simulink model "model_cnn"  (R2020a)
settings: Solver=VariableStepAuto  StartTime=0.0  StopTime=1e6/fs  RelTol=1e-3
PreLoadFcn:
  | setup_imports;
  | %dense2_numerictype = fixdt(1,18,10);
  | %conv1_numerictype = fixdt(1,18,21);
InitFcn:
  | % Intermediate signal dimensions
  | input_dim = [1, 2, 128];
  | layer1_dim = hInterConvLayerDims([1,3,1,64],input_dim,1); % dims : [C,H,W]
  | layer2_dim = hInterConvLayerDims([2,3,64,16],layer1_dim,1);% dims : [C,H,W]
  | layer3_dim = [1,128];
  | 
  | % Conv Layer 1 dimensions
  | conv1_dims = struct(...
  |     'input_dim',    input_dim,...       input_dim = C,H,W
  |     'filter_dim',   [1, 3, 1, 64],...  filter_dim = K,J,C,N
  |     'stride',       1,...
  |     'row_output',   3,...
  |     'output_dim',   layer1_dim);
  | 
  | % Conv Layer 2 dimensions
  | conv2_dims = struct(...
  |     'input_dim',    layer1_dim,...      input = C,H.W
  |     'filter_dim',   [2, 3, 64, 16],...  filter_dim = K,J,C,N
  |     'stride',       1,...
  |     'row_output',   2*3*64,...
  |     'output_dim',   layer2_dim);
  | 
  | % Dense Layer 1 dimensions
  | dense1_dims = struct(...
  |     'input_dim',    layer2_dim,...      input = C,H,W
  |     'weight_dim',   [1984, 128],...     weight_dim = H,W
  |     'output_dim',   layer3_dim);
  | 
  | % Load saved weights and input
  | setup_imports;
  | 
  | fs = 128e6;
  | fs_axi = 100e6;
  | R = 32;
values from neighbouring files (symbols this model uses):
  datatypeInput = X_test.numerictype    [setup_imports.m]
  gemm_wconv1 = fi(hInterleaveFilters(Wconv1),1,16)    [setup_imports.m]
  gemm_wconv2 = fi(hInterleaveFilters(Wconv2),1,16)    [setup_imports.m]
  wdense1 = fi(Wdense1,1,16)    [setup_imports.m]
  wdense2 = fi(Wdense2,1,16)    [setup_imports.m]
undefined symbols (not defined in the file or in its folder): ltehdlRAMinitPO2
libraries: hdlsllib x1022, dspsigops x3, dspsrcs4 x2
(part 2 of 23)

== system model_cnn/HDL CNN Model/Conv Layer 2/Vector Slice Selection ==
  frameIn : Inport
  validIn : Inport  Port=2
  Frame Slicer : MATLAB Function  TreatAsAtomicUnit=on
  Frame Slicer1 : MATLAB Function  TreatAsAtomicUnit=on
  Frame Slicer2 : MATLAB Function  TreatAsAtomicUnit=on
  Frame Slicer3 : MATLAB Function  TreatAsAtomicUnit=on
  HDL Counter : hdlsllib/Sources/HDL Counter  CountType=Count limited  CountInit=0  CountStep=1  CountMax=3  CountFromType=Initial value  CountFrom=0  CountResetPort=off  CountLoadPort=off  CountEnbPort=on  CountDirPort=off  CountDataType=Unsigned  CountWordLen=2  CountFracLen=0  CountSampTime=1
  Multiport Switch : MultiPortSwitch  DataPortOrder=Zero-based contiguous  Inputs=4  DiagnosticForDefault=None  zeroidx=on
  frameOut : Outport
  validOut : Outport  Port=2
  wires:
  frameIn/1 -> Frame Slicer/1(frameIn), Frame Slicer3/1(frameIn), Frame Slicer2/1(frameIn), Frame Slicer1/1(frameIn)
  validIn/1 -> validOut/1, HDL Counter/1
  HDL Counter/1 -> Multiport Switch/1
  Frame Slicer/1(slicedFrame) -> Multiport Switch/2
  Frame Slicer1/1(slicedFrame) -> Multiport Switch/3
  Frame Slicer2/1(slicedFrame) -> Multiport Switch/4
  Frame Slicer3/1(slicedFrame) -> Multiport Switch/5
  Multiport Switch/1 -> frameOut/1

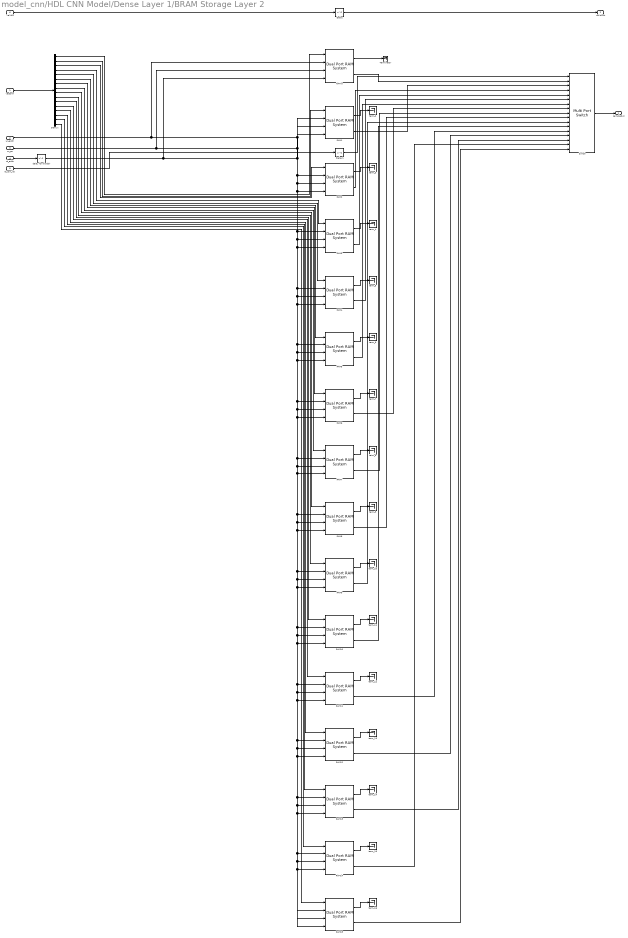
== system model_cnn/HDL CNN Model/Dense Layer 1/BRAM Storage Layer 2 ==
  vectorIn : Inport
  wr_addr : Inport  Port=2
  wr_en : Inport  Port=3
  rd_addr : Inport  Port=4
  rd_row_idx : Inport  Port=5
  validIn : Inport  Port=6
  Delay : Delay
  Delay1 : Delay
  Demux : Demux  Outputs=16
  RAM 0 : hdlsllib/HDL RAMs/Dual Port RAM System  RAMType=Dual port  WriteOutputValue=New data  RAMInitialValue=0  SimulateUsing=Code generation
      settings: SourceProductBaseCode=SL
  RAM{1..15} (15 alike) : hdlsllib/HDL RAMs/Dual Port RAM System  RAMType=Dual port  WriteOutputValue=New data  RAMInitialValue=0  SimulateUsing=Code generation
      settings: SourceProductBaseCode=SL
  Switch : MultiPortSwitch  DataPortOrder=Zero-based contiguous  Inputs=16  zeroidx=on
  Terminator : Terminator
  delay for rd addr : Delay  DelayLength=1
  term_{2..16} (15 alike) : Terminator
  sampleOut : Outport
  validOut : Outport  Port=2
  wires:
  vectorIn/1 -> Demux/1  "vectorIn"
  Demux/1 -> RAM 0/1
  Switch/1 -> sampleOut/1  "fff_sampleOut"
  wr_addr/1 -> RAM15/2, RAM14/2, RAM13/2, RAM12/2, RAM11/2, RAM10/2, RAM9/2, RAM8/2, RAM7/2, RAM6/2, RAM5/2, RAM4/2, RAM3/2, RAM2/2, RAM1/2, RAM 0/2  "wr_addr"
  RAM 0/1 -> Terminator/1
  RAM 0/2 -> Switch/2  "ram_out"
  validIn/1 -> Delay/1  "vvv valid"
  Delay/1 -> validOut/1  "fff_valid"
  wr_en/1 -> RAM15/3, RAM14/3, RAM13/3, RAM12/3, RAM11/3, RAM10/3, RAM9/3, RAM8/3, RAM7/3, RAM6/3, RAM5/3, RAM4/3, RAM3/3, RAM2/3, RAM1/3, RAM 0/3  "wr_en"
  rd_addr/1 -> delay for rd addr/1  "fff_rd_addr"
  Demux/2 -> RAM1/1
  RAM1/2 -> Switch/3  "fff_rd_row_2"
  RAM1/1 -> term_2/1
  Demux/3 -> RAM2/1
  RAM2/2 -> Switch/4
  RAM2/1 -> term_3/1
  Demux/4 -> RAM3/1
  RAM3/2 -> Switch/5
  RAM3/1 -> term_4/1
  Demux/5 -> RAM4/1
  RAM4/2 -> Switch/6
  RAM4/1 -> term_5/1
  Demux/6 -> RAM5/1  "vvv"
  RAM5/2 -> Switch/7
  RAM5/1 -> term_6/1
  Demux/7 -> RAM6/1
  RAM6/2 -> Switch/8
  RAM6/1 -> term_7/1
  Demux/8 -> RAM7/1
  RAM7/2 -> Switch/9
  RAM7/1 -> term_8/1
  Demux/9 -> RAM8/1
  RAM8/2 -> Switch/10
  RAM8/1 -> term_9/1
  Demux/10 -> RAM9/1
  RAM9/2 -> Switch/11
  RAM9/1 -> term_10/1
  Demux/11 -> RAM10/1
  RAM10/2 -> Switch/12
  RAM10/1 -> term_11/1
  Demux/12 -> RAM11/1
  RAM11/2 -> Switch/13
  RAM11/1 -> term_12/1
  Demux/13 -> RAM12/1
  RAM12/2 -> Switch/14
  RAM12/1 -> term_13/1
  Demux/14 -> RAM13/1
  RAM13/2 -> Switch/15
  RAM13/1 -> term_14/1
  Demux/15 -> RAM14/1
  RAM14/2 -> Switch/16
  RAM14/1 -> term_15/1
  Demux/16 -> RAM15/1
  RAM15/2 -> Switch/17  "valueOut"
  RAM15/1 -> term_16/1
  rd_row_idx/1 -> Delay1/1
  Delay1/1 -> Switch/1  "fff_rd_row"
  delay for rd addr/1 -> RAM15/4, RAM14/4, RAM13/4, RAM12/4, RAM11/4, RAM10/4, RAM9/4, RAM8/4, RAM7/4, RAM6/4, RAM5/4, RAM4/4, RAM3/4, RAM2/4, RAM1/4, RAM 0/4

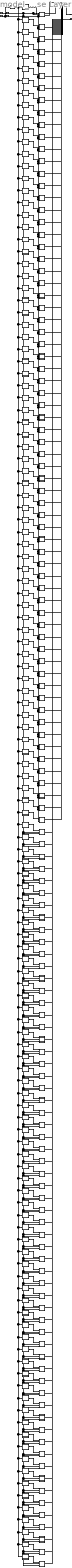
== system model_cnn/HDL CNN Model/Dense Layer 1/Dense Layer 1 ==
  dataIn : Inport
  valid : Inport  Port=2
  Delay : Delay  DelayLength=1
  Delay1 : Delay  DelayLength=1
  HDL Counter : hdlsllib/Sources/HDL Counter  CountType=Count limited  CountInit=0  CountStep=1  CountMax=1984-1  CountFromType=Initial value  CountFrom=0  CountResetPort=off  CountLoadPort=off  CountEnbPort=on  CountDirPort=off  CountDataType=Unsigned  CountWordLen=ceil(log2(1984))  CountFracLen=0  CountSampTime=1
  Vector Concatenate : Concatenate  NumInputs=128
  Weight Storage 0 : Subsystem  mask{dim=1}
      mask prompts: dim "Filter Selection"
  Weight Storage1 : Subsystem  mask{dim=2}
      mask prompts: dim "Filter Selection"
  Weight Storage10 : Subsystem  mask{dim=11}
      mask prompts: dim "Filter Selection"
  Weight Storage100 : Subsystem  mask{dim=101}
      mask prompts: dim "Filter Selection"
  Weight Storage101 : Subsystem  mask{dim=102}
      mask prompts: dim "Filter Selection"
  Weight Storage102 : Subsystem  mask{dim=103}
      mask prompts: dim "Filter Selection"
  Weight Storage103 : Subsystem  mask{dim=104}
      mask prompts: dim "Filter Selection"
  Weight Storage104 : Subsystem  mask{dim=105}
      mask prompts: dim "Filter Selection"
  Weight Storage105 : Subsystem  mask{dim=106}
      mask prompts: dim "Filter Selection"
  Weight Storage106 : Subsystem  mask{dim=107}
      mask prompts: dim "Filter Selection"
  Weight Storage107 : Subsystem  mask{dim=108}
      mask prompts: dim "Filter Selection"
  Weight Storage108 : Subsystem  mask{dim=109}
      mask prompts: dim "Filter Selection"
  Weight Storage109 : Subsystem  mask{dim=110}
      mask prompts: dim "Filter Selection"
  Weight Storage11 : Subsystem  mask{dim=12}
      mask prompts: dim "Filter Selection"
  Weight Storage110 : Subsystem  mask{dim=111}
      mask prompts: dim "Filter Selection"
  Weight Storage111 : Subsystem  mask{dim=112}
      mask prompts: dim "Filter Selection"
  Weight Storage112 : Subsystem  mask{dim=113}
      mask prompts: dim "Filter Selection"
  Weight Storage113 : Subsystem  mask{dim=114}
      mask prompts: dim "Filter Selection"
  Weight Storage114 : Subsystem  mask{dim=115}
      mask prompts: dim "Filter Selection"
  Weight Storage115 : Subsystem  mask{dim=116}
      mask prompts: dim "Filter Selection"
  Weight Storage116 : Subsystem  mask{dim=117}
      mask prompts: dim "Filter Selection"
  Weight Storage117 : Subsystem  mask{dim=118}
      mask prompts: dim "Filter Selection"
  Weight Storage118 : Subsystem  mask{dim=119}
      mask prompts: dim "Filter Selection"
  Weight Storage119 : Subsystem  mask{dim=120}
      mask prompts: dim "Filter Selection"
  Weight Storage12 : Subsystem  mask{dim=13}
      mask prompts: dim "Filter Selection"
  Weight Storage120 : Subsystem  mask{dim=121}
      mask prompts: dim "Filter Selection"
  Weight Storage121 : Subsystem  mask{dim=122}
      mask prompts: dim "Filter Selection"
  Weight Storage122 : Subsystem  mask{dim=123}
      mask prompts: dim "Filter Selection"
  Weight Storage123 : Subsystem  mask{dim=124}
      mask prompts: dim "Filter Selection"
  Weight Storage124 : Subsystem  mask{dim=125}
      mask prompts: dim "Filter Selection"
  Weight Storage125 : Subsystem  mask{dim=126}
      mask prompts: dim "Filter Selection"
  Weight Storage126 : Subsystem  mask{dim=127}
      mask prompts: dim "Filter Selection"
  Weight Storage127 : Subsystem  mask{dim=128}
      mask prompts: dim "Filter Selection"
  Weight Storage13 : Subsystem  mask{dim=14}
      mask prompts: dim "Filter Selection"
  Weight Storage14 : Subsystem  mask{dim=15}
      mask prompts: dim "Filter Selection"
  Weight Storage15 : Subsystem  mask{dim=16}
      mask prompts: dim "Filter Selection"
  Weight Storage16 : Subsystem  mask{dim=17}
      mask prompts: dim "Filter Selection"
  Weight Storage17 : Subsystem  mask{dim=18}
      mask prompts: dim "Filter Selection"
  Weight Storage18 : Subsystem  mask{dim=19}
      mask prompts: dim "Filter Selection"
  Weight Storage19 : Subsystem  mask{dim=20}
      mask prompts: dim "Filter Selection"
  Weight Storage2 : Subsystem  mask{dim=3}
      mask prompts: dim "Filter Selection"
  Weight Storage20 : Subsystem  mask{dim=21}
      mask prompts: dim "Filter Selection"
  Weight Storage21 : Subsystem  mask{dim=22}
      mask prompts: dim "Filter Selection"
  Weight Storage22 : Subsystem  mask{dim=23}
      mask prompts: dim "Filter Selection"
  Weight Storage23 : Subsystem  mask{dim=24}
      mask prompts: dim "Filter Selection"
  Weight Storage24 : Subsystem  mask{dim=25}
      mask prompts: dim "Filter Selection"
  Weight Storage25 : Subsystem  mask{dim=26}
      mask prompts: dim "Filter Selection"
  Weight Storage26 : Subsystem  mask{dim=27}
      mask prompts: dim "Filter Selection"
  Weight Storage27 : Subsystem  mask{dim=28}
      mask prompts: dim "Filter Selection"
  Weight Storage28 : Subsystem  mask{dim=29}
      mask prompts: dim "Filter Selection"
  Weight Storage29 : Subsystem  mask{dim=30}
      mask prompts: dim "Filter Selection"
  Weight Storage3 : Subsystem  mask{dim=4}
      mask prompts: dim "Filter Selection"
  Weight Storage30 : Subsystem  mask{dim=31}
      mask prompts: dim "Filter Selection"
  Weight Storage31 : Subsystem  mask{dim=32}
      mask prompts: dim "Filter Selection"
  Weight Storage32 : Subsystem  mask{dim=33}
      mask prompts: dim "Filter Selection"
  Weight Storage33 : Subsystem  mask{dim=34}
      mask prompts: dim "Filter Selection"
  Weight Storage34 : Subsystem  mask{dim=35}
      mask prompts: dim "Filter Selection"
  Weight Storage35 : Subsystem  mask{dim=36}
      mask prompts: dim "Filter Selection"
  Weight Storage36 : Subsystem  mask{dim=37}
      mask prompts: dim "Filter Selection"
  Weight Storage37 : Subsystem  mask{dim=38}
      mask prompts: dim "Filter Selection"
  Weight Storage38 : Subsystem  mask{dim=39}
      mask prompts: dim "Filter Selection"
  Weight Storage39 : Subsystem  mask{dim=40}
      mask prompts: dim "Filter Selection"
  Weight Storage4 : Subsystem  mask{dim=5}
      mask prompts: dim "Filter Selection"
  Weight Storage40 : Subsystem  mask{dim=41}
      mask prompts: dim "Filter Selection"
  Weight Storage41 : Subsystem  mask{dim=42}
      mask prompts: dim "Filter Selection"
  Weight Storage42 : Subsystem  mask{dim=43}
      mask prompts: dim "Filter Selection"
  Weight Storage43 : Subsystem  mask{dim=44}
      mask prompts: dim "Filter Selection"
  Weight Storage44 : Subsystem  mask{dim=45}
      mask prompts: dim "Filter Selection"
  Weight Storage45 : Subsystem  mask{dim=46}
      mask prompts: dim "Filter Selection"
  Weight Storage46 : Subsystem  mask{dim=47}
      mask prompts: dim "Filter Selection"
  Weight Storage47 : Subsystem  mask{dim=48}
      mask prompts: dim "Filter Selection"
  Weight Storage48 : Subsystem  mask{dim=49}
      mask prompts: dim "Filter Selection"
  Weight Storage49 : Subsystem  mask{dim=50}
      mask prompts: dim "Filter Selection"
  Weight Storage5 : Subsystem  mask{dim=6}
      mask prompts: dim "Filter Selection"
  Weight Storage50 : Subsystem  mask{dim=51}
      mask prompts: dim "Filter Selection"
  Weight Storage51 : Subsystem  mask{dim=52}
      mask prompts: dim "Filter Selection"
  Weight Storage52 : Subsystem  mask{dim=53}
      mask prompts: dim "Filter Selection"
  Weight Storage53 : Subsystem  mask{dim=54}
      mask prompts: dim "Filter Selection"
  Weight Storage54 : Subsystem  mask{dim=55}
      mask prompts: dim "Filter Selection"
  Weight Storage55 : Subsystem  mask{dim=56}
      mask prompts: dim "Filter Selection"
  Weight Storage56 : Subsystem  mask{dim=57}
      mask prompts: dim "Filter Selection"
  Weight Storage57 : Subsystem  mask{dim=58}
      mask prompts: dim "Filter Selection"
  Weight Storage58 : Subsystem  mask{dim=59}
      mask prompts: dim "Filter Selection"
  Weight Storage59 : Subsystem  mask{dim=60}
      mask prompts: dim "Filter Selection"
  Weight Storage6 : Subsystem  mask{dim=7}
      mask prompts: dim "Filter Selection"
  Weight Storage60 : Subsystem  mask{dim=61}
      mask prompts: dim "Filter Selection"
  Weight Storage61 : Subsystem  mask{dim=62}
      mask prompts: dim "Filter Selection"
  Weight Storage62 : Subsystem  mask{dim=63}
      mask prompts: dim "Filter Selection"
  Weight Storage63 : Subsystem  mask{dim=64}
      mask prompts: dim "Filter Selection"
  Weight Storage64 : Subsystem  mask{dim=65}
      mask prompts: dim "Filter Selection"
  Weight Storage65 : Subsystem  mask{dim=66}
      mask prompts: dim "Filter Selection"
  Weight Storage66 : Subsystem  mask{dim=67}
      mask prompts: dim "Filter Selection"
  Weight Storage67 : Subsystem  mask{dim=68}
      mask prompts: dim "Filter Selection"
  Weight Storage68 : Subsystem  mask{dim=69}
      mask prompts: dim "Filter Selection"
  Weight Storage69 : Subsystem  mask{dim=70}
      mask prompts: dim "Filter Selection"
  Weight Storage7 : Subsystem  mask{dim=8}
      mask prompts: dim "Filter Selection"
  Weight Storage70 : Subsystem  mask{dim=71}
      mask prompts: dim "Filter Selection"
  Weight Storage71 : Subsystem  mask{dim=72}
      mask prompts: dim "Filter Selection"
  Weight Storage72 : Subsystem  mask{dim=73}
      mask prompts: dim "Filter Selection"
  Weight Storage73 : Subsystem  mask{dim=74}
      mask prompts: dim "Filter Selection"
  Weight Storage74 : Subsystem  mask{dim=75}
      mask prompts: dim "Filter Selection"
  Weight Storage75 : Subsystem  mask{dim=76}
      mask prompts: dim "Filter Selection"
  Weight Storage76 : Subsystem  mask{dim=77}
      mask prompts: dim "Filter Selection"
  Weight Storage77 : Subsystem  mask{dim=78}
      mask prompts: dim "Filter Selection"
  Weight Storage78 : Subsystem  mask{dim=79}
      mask prompts: dim "Filter Selection"
  Weight Storage79 : Subsystem  mask{dim=80}
      mask prompts: dim "Filter Selection"
  Weight Storage8 : Subsystem  mask{dim=9}
      mask prompts: dim "Filter Selection"
  Weight Storage80 : Subsystem  mask{dim=81}
      mask prompts: dim "Filter Selection"
  Weight Storage81 : Subsystem  mask{dim=82}
      mask prompts: dim "Filter Selection"
  Weight Storage82 : Subsystem  mask{dim=83}
      mask prompts: dim "Filter Selection"
  Weight Storage83 : Subsystem  mask{dim=84}
      mask prompts: dim "Filter Selection"
  Weight Storage84 : Subsystem  mask{dim=85}
      mask prompts: dim "Filter Selection"
  Weight Storage85 : Subsystem  mask{dim=86}
      mask prompts: dim "Filter Selection"
  Weight Storage86 : Subsystem  mask{dim=87}
      mask prompts: dim "Filter Selection"
  Weight Storage87 : Subsystem  mask{dim=88}
      mask prompts: dim "Filter Selection"
  Weight Storage88 : Subsystem  mask{dim=89}
      mask prompts: dim "Filter Selection"
  Weight Storage89 : Subsystem  mask{dim=90}
      mask prompts: dim "Filter Selection"
  Weight Storage9 : Subsystem  mask{dim=10}
      mask prompts: dim "Filter Selection"
  Weight Storage90 : Subsystem  mask{dim=91}
      mask prompts: dim "Filter Selection"
  Weight Storage91 : Subsystem  mask{dim=92}
      mask prompts: dim "Filter Selection"
  Weight Storage92 : Subsystem  mask{dim=93}
      mask prompts: dim "Filter Selection"
  Weight Storage93 : Subsystem  mask{dim=94}
      mask prompts: dim "Filter Selection"
  Weight Storage94 : Subsystem  mask{dim=95}
      mask prompts: dim "Filter Selection"
  Weight Storage95 : Subsystem  mask{dim=96}
      mask prompts: dim "Filter Selection"
  Weight Storage96 : Subsystem  mask{dim=97}
      mask prompts: dim "Filter Selection"
  Weight Storage97 : Subsystem  mask{dim=98}
      mask prompts: dim "Filter Selection"
  Weight Storage98 : Subsystem  mask{dim=99}
      mask prompts: dim "Filter Selection"
  Weight Storage99 : Subsystem  mask{dim=100}
      mask prompts: dim "Filter Selection"
  adder 0 : Subsystem
  adder1 : Subsystem
  adder10 : Subsystem
  adder100 : Subsystem
  adder101 : Subsystem
  adder102 : Subsystem
  adder103 : Subsystem
  adder104 : Subsystem
  adder105 : Subsystem
  adder106 : Subsystem
  adder107 : Subsystem
  adder108 : Subsystem
  adder109 : Subsystem
  adder11 : Subsystem
  adder110 : Subsystem
  adder111 : Subsystem
  adder112 : Subsystem
  adder113 : Subsystem
  adder114 : Subsystem
  adder115 : Subsystem
  adder116 : Subsystem
  adder117 : Subsystem
  adder118 : Subsystem
  adder119 : Subsystem
  adder12 : Subsystem
  adder120 : Subsystem
  adder121 : Subsystem
  adder122 : Subsystem
  adder123 : Subsystem
  adder124 : Subsystem
  adder125 : Subsystem
  adder126 : Subsystem
  adder127 : Subsystem
  adder13 : Subsystem
  adder14 : Subsystem
  adder15 : Subsystem
  adder16 : Subsystem
  adder17 : Subsystem
  adder18 : Subsystem
  adder19 : Subsystem
  adder2 : Subsystem
  adder20 : Subsystem
  adder21 : Subsystem
  adder22 : Subsystem
  adder23 : Subsystem
  adder24 : Subsystem
  adder25 : Subsystem
  adder26 : Subsystem
  adder27 : Subsystem
  adder28 : Subsystem
  adder29 : Subsystem
  adder3 : Subsystem
  adder30 : Subsystem
  adder31 : Subsystem
  adder32 : Subsystem
  adder33 : Subsystem
  adder34 : Subsystem
  adder35 : Subsystem
  adder36 : Subsystem
  adder37 : Subsystem
  adder38 : Subsystem
  adder39 : Subsystem
  adder4 : Subsystem
  adder40 : Subsystem
  adder41 : Subsystem
  adder42 : Subsystem
  adder43 : Subsystem
  adder44 : Subsystem
  adder45 : Subsystem
  adder46 : Subsystem
  adder47 : Subsystem
  adder48 : Subsystem
  adder49 : Subsystem
  adder5 : Subsystem
  adder50 : Subsystem
  adder51 : Subsystem
  adder52 : Subsystem
  adder53 : Subsystem
  adder54 : Subsystem
  adder55 : Subsystem
  adder56 : Subsystem
  adder57 : Subsystem
  adder58 : Subsystem
  adder59 : Subsystem
  adder6 : Subsystem
  adder60 : Subsystem
  adder61 : Subsystem
  adder62 : Subsystem
  adder63 : Subsystem
  adder64 : Subsystem
  adder65 : Subsystem
  adder66 : Subsystem
  adder67 : Subsystem
  adder68 : Subsystem
  adder69 : Subsystem
  adder7 : Subsystem
  adder70 : Subsystem
  adder71 : Subsystem
  adder72 : Subsystem
  adder73 : Subsystem
  adder74 : Subsystem
  adder75 : Subsystem
  adder76 : Subsystem
  adder77 : Subsystem
  adder78 : Subsystem
  adder79 : Subsystem
  adder8 : Subsystem
  adder80 : Subsystem
  adder81 : Subsystem
  adder82 : Subsystem
  adder83 : Subsystem
  adder84 : Subsystem
  adder85 : Subsystem
  adder86 : Subsystem
  adder87 : Subsystem
  adder88 : Subsystem
  adder89 : Subsystem
  adder9 : Subsystem
  adder90 : Subsystem
  adder91 : Subsystem
  adder92 : Subsystem
  adder93 : Subsystem
  adder94 : Subsystem
  adder95 : Subsystem
  adder96 : Subsystem
  adder97 : Subsystem
  adder98 : Subsystem
  adder99 : Subsystem
  dataOut : Outport
  validOut : Outport  Port=2
  wires:
  dataIn/1 -> Delay/1
  valid/1 -> HDL Counter/1, Delay1/1
  HDL Counter/1 -> Weight Storage126/1(count_Weights), Weight Storage127/1(count_Weights), Weight Storage125/1(count_Weights), Weight Storage124/1(count_Weights), Weight Storage123/1(count_Weights), Weight Storage122/1(count_Weights), Weight Storage121/1(count_Weights), Weight Storage120/1(count_Weights), Weight Storage119/1(count_Weights), Weight Storage118/1(count_Weights), Weight Storage117/1(count_Weights), Weight Storage116/1(count_Weights), Weight Storage115/1(count_Weights), Weight Storage114/1(count_Weights), Weight Storage113/1(count_Weights), Weight Storage112/1(count_Weights), Weight Storage111/1(count_Weights), Weight Storage110/1(count_Weights), Weight Storage109/1(count_Weights), Weight Storage108/1(count_Weights), Weight Storage107/1(count_Weights), Weight Storage106/1(count_Weights), Weight Storage105/1(count_Weights), Weight Storage104/1(count_Weights), Weight Storage103/1(count_Weights), Weight Storage102/1(count_Weights), Weight Storage101/1(count_Weights), Weight Storage100/1(count_Weights), Weight Storage99/1(count_Weights), Weight Storage98/1(count_Weights), Weight Storage97/1(count_Weights), Weight Storage96/1(count_Weights), Weight Storage95/1(count_Weights), Weight Storage94/1(count_Weights), Weight Storage93/1(count_Weights), Weight Storage92/1(count_Weights), Weight Storage91/1(count_Weights), Weight Storage90/1(count_Weights), Weight Storage89/1(count_Weights), Weight Storage88/1(count_Weights), Weight Storage87/1(count_Weights), Weight Storage86/1(count_Weights), Weight Storage85/1(count_Weights), Weight Storage84/1(count_Weights), Weight Storage83/1(count_Weights), Weight Storage82/1(count_Weights), Weight Storage81/1(count_Weights), Weight Storage80/1(count_Weights), Weight Storage79/1(count_Weights), Weight Storage78/1(count_Weights), Weight Storage77/1(count_Weights), Weight Storage76/1(count_Weights), Weight Storage75/1(count_Weights), Weight Storage74/1(count_Weights), Weight Storage73/1(count_Weights), Weight Storage72/1(count_Weights), Weight Storage71/1(count_Weights), Weight Storage70/1(count_Weights), Weight Storage69/1(count_Weights), Weight Storage68/1(count_Weights), Weight Storage67/1(count_Weights), Weight Storage66/1(count_Weights), Weight Storage65/1(count_Weights), Weight Storage64/1(count_Weights), Weight Storage63/1(count_Weights), Weight Storage62/1(count_Weights), Weight Storage61/1(count_Weights), Weight Storage60/1(count_Weights), Weight Storage59/1(count_Weights), Weight Storage58/1(count_Weights), Weight Storage57/1(count_Weights), Weight Storage56/1(count_Weights), Weight Storage55/1(count_Weights), Weight Storage54/1(count_Weights), Weight Storage53/1(count_Weights), Weight Storage52/1(count_Weights), Weight Storage51/1(count_Weights), Weight Storage50/1(count_Weights), Weight Storage49/1(count_Weights), Weight Storage48/1(count_Weights), Weight Storage47/1(count_Weights), Weight Storage46/1(count_Weights), Weight Storage45/1(count_Weights), Weight Storage44/1(count_Weights), Weight Storage43/1(count_Weights), Weight Storage42/1(count_Weights), Weight Storage41/1(count_Weights), Weight Storage40/1(count_Weights), Weight Storage39/1(count_Weights), Weight Storage38/1(count_Weights), Weight Storage37/1(count_Weights), Weight Storage36/1(count_Weights), Weight Storage35/1(count_Weights), Weight Storage34/1(count_Weights), Weight Storage33/1(count_Weights), Weight Storage32/1(count_Weights), Weight Storage31/1(count_Weights), Weight Storage30/1(count_Weights), Weight Storage29/1(count_Weights), Weight Storage28/1(count_Weights), Weight Storage27/1(count_Weights), Weight Storage26/1(count_Weights), Weight Storage25/1(count_Weights), Weight Storage24/1(count_Weights), Weight Storage23/1(count_Weights), Weight Storage22/1(count_Weights), Weight Storage21/1(count_Weights), Weight Storage20/1(count_Weights), Weight Storage19/1(count_Weights), Weight Storage18/1(count_Weights), Weight Storage17/1(count_Weights), Weight Storage16/1(count_Weights), Weight Storage15/1(count_Weights), Weight Storage14/1(count_Weights), Weight Storage13/1(count_Weights), Weight Storage12/1(count_Weights), Weight Storage11/1(count_Weights), Weight Storage10/1(count_Weights), Weight Storage9/1(count_Weights), Weight Storage8/1(count_Weights), Weight Storage7/1(count_Weights), Weight Storage6/1(count_Weights), Weight Storage5/1(count_Weights), Weight Storage4/1(count_Weights), Weight Storage3/1(count_Weights), Weight Storage2/1(count_Weights), Weight Storage1/1(count_Weights), Weight Storage 0/1(count_Weights)  "count_Weights"
  Vector Concatenate/1 -> dataOut/1  "dataOut"
  Weight Storage 0/1(Out1) -> adder 0/1(In1)  "weight"
  Delay1/1 -> adder126/3(In3), adder127/3(In3), adder125/3(In3), adder124/3(In3), adder123/3(In3), adder122/3(In3), adder121/3(In3), adder120/3(In3), adder119/3(In3), adder118/3(In3), adder117/3(In3), adder116/3(In3), adder115/3(In3), adder114/3(In3), adder113/3(In3), adder112/3(In3), adder111/3(In3), adder110/3(In3), adder109/3(In3), adder108/3(In3), adder107/3(In3), adder106/3(In3), adder105/3(In3), adder104/3(In3), adder103/3(In3), adder102/3(In3), adder101/3(In3), adder100/3(In3), adder99/3(In3), adder98/3(In3), adder97/3(In3), adder96/3(In3), adder95/3(In3), adder94/3(In3), adder93/3(In3), adder92/3(In3), adder91/3(In3), adder90/3(In3), adder89/3(In3), adder88/3(In3), adder87/3(In3), adder86/3(In3), adder85/3(In3), adder84/3(In3), adder83/3(In3), adder82/3(In3), adder81/3(In3), adder80/3(In3), adder79/3(In3), adder78/3(In3), adder77/3(In3), adder76/3(In3), adder75/3(In3), adder74/3(In3), adder73/3(In3), adder72/3(In3), adder71/3(In3), adder70/3(In3), adder69/3(In3), adder68/3(In3), adder67/3(In3), adder65/3(In3), adder66/3(In3), adder64/3(In3), adder63/3(In3), adder62/3(In3), adder61/3(In3), adder60/3(In3), adder59/3(In3), adder58/3(In3), adder57/3(In3), adder56/3(In3), adder55/3(In3), adder54/3(In3), adder53/3(In3), adder52/3(In3), adder51/3(In3), adder50/3(In3), adder49/3(In3), adder48/3(In3), adder47/3(In3), adder46/3(In3), adder45/3(In3), adder44/3(In3), adder43/3(In3), adder42/3(In3), adder41/3(In3), adder40/3(In3), adder39/3(In3), adder38/3(In3), adder37/3(In3), adder36/3(In3), adder35/3(In3), adder34/3(In3), adder33/3(In3), adder32/3(In3), adder31/3(In3), adder30/3(In3), adder29/3(In3), adder28/3(In3), adder27/3(In3), adder26/3(In3), adder25/3(In3), adder24/3(In3), adder23/3(In3), adder22/3(In3), adder21/3(In3), adder20/3(In3), adder19/3(In3), adder18/3(In3), adder17/3(In3), adder16/3(In3), adder15/3(In3), adder14/3(In3), adder13/3(In3), adder12/3(In3), adder11/3(In3), adder10/3(In3), adder9/3(In3), adder8/3(In3), adder7/3(In3), adder6/3(In3), adder5/3(In3), adder4/3(In3), adder3/3(In3), adder2/3(In3), adder1/3(In3), adder 0/3(In3)  "valid"
  adder 0/2(validOut) -> validOut/1  "validOut"
  adder 0/1(dataOut) -> Vector Concatenate/1
  Weight Storage1/1(Out1) -> adder1/1(In1)
  adder1/1(dataOut) -> Vector Concatenate/2
  Weight Storage2/1(Out1) -> adder2/1(In1)
  adder2/1(dataOut) -> Vector Concatenate/3
  Weight Storage3/1(Out1) -> adder3/1(In1)
  adder3/1(dataOut) -> Vector Concatenate/4
  Weight Storage4/1(Out1) -> adder4/1(In1)
  adder4/1(dataOut) -> Vector Concatenate/5
  Weight Storage5/1(Out1) -> adder5/1(In1)
  adder5/1(dataOut) -> Vector Concatenate/6
  Weight Storage6/1(Out1) -> adder6/1(In1)
  adder6/1(dataOut) -> Vector Concatenate/7
  Weight Storage7/1(Out1) -> adder7/1(In1)
  adder7/1(dataOut) -> Vector Concatenate/8
  Weight Storage8/1(Out1) -> adder8/1(In1)
  adder8/1(dataOut) -> Vector Concatenate/9
  Weight Storage9/1(Out1) -> adder9/1(In1)
  adder9/1(dataOut) -> Vector Concatenate/10
  Weight Storage10/1(Out1) -> adder10/1(In1)
  adder10/1(dataOut) -> Vector Concatenate/11
  Weight Storage11/1(Out1) -> adder11/1(In1)
  adder11/1(dataOut) -> Vector Concatenate/12
  Weight Storage12/1(Out1) -> adder12/1(In1)
  adder12/1(dataOut) -> Vector Concatenate/13
  Weight Storage13/1(Out1) -> adder13/1(In1)
  adder13/1(dataOut) -> Vector Concatenate/14
  Weight Storage14/1(Out1) -> adder14/1(In1)
  adder14/1(dataOut) -> Vector Concatenate/15
  Weight Storage15/1(Out1) -> adder15/1(In1)
  adder15/1(dataOut) -> Vector Concatenate/16
  Weight Storage16/1(Out1) -> adder16/1(In1)
  adder16/1(dataOut) -> Vector Concatenate/17
  Weight Storage17/1(Out1) -> adder17/1(In1)
  adder17/1(dataOut) -> Vector Concatenate/18
  Weight Storage18/1(Out1) -> adder18/1(In1)
  adder18/1(dataOut) -> Vector Concatenate/19
  Weight Storage19/1(Out1) -> adder19/1(In1)
  adder19/1(dataOut) -> Vector Concatenate/20
  Weight Storage20/1(Out1) -> adder20/1(In1)
  adder20/1(dataOut) -> Vector Concatenate/21
  Weight Storage21/1(Out1) -> adder21/1(In1)
  adder21/1(dataOut) -> Vector Concatenate/22
  Weight Storage22/1(Out1) -> adder22/1(In1)
  adder22/1(dataOut) -> Vector Concatenate/23
  Weight Storage23/1(Out1) -> adder23/1(In1)
  adder23/1(dataOut) -> Vector Concatenate/24
  Weight Storage24/1(Out1) -> adder24/1(In1)
  adder24/1(dataOut) -> Vector Concatenate/25
  Weight Storage25/1(Out1) -> adder25/1(In1)
  adder25/1(dataOut) -> Vector Concatenate/26
  Weight Storage26/1(Out1) -> adder26/1(In1)
  adder26/1(dataOut) -> Vector Concatenate/27
  Weight Storage27/1(Out1) -> adder27/1(In1)
  adder27/1(dataOut) -> Vector Concatenate/28
  Weight Storage28/1(Out1) -> adder28/1(In1)
  adder28/1(dataOut) -> Vector Concatenate/29
  Weight Storage29/1(Out1) -> adder29/1(In1)
  adder29/1(dataOut) -> Vector Concatenate/30
  Weight Storage30/1(Out1) -> adder30/1(In1)
  adder30/1(dataOut) -> Vector Concatenate/31
  Weight Storage31/1(Out1) -> adder31/1(In1)
  adder31/1(dataOut) -> Vector Concatenate/32
  Weight Storage32/1(Out1) -> adder32/1(In1)
  adder32/1(dataOut) -> Vector Concatenate/33
  Weight Storage33/1(Out1) -> adder33/1(In1)
  adder33/1(dataOut) -> Vector Concatenate/34
  Weight Storage34/1(Out1) -> adder34/1(In1)
  adder34/1(dataOut) -> Vector Concatenate/35
  Weight Storage35/1(Out1) -> adder35/1(In1)
  adder35/1(dataOut) -> Vector Concatenate/36
  Weight Storage36/1(Out1) -> adder36/1(In1)
  adder36/1(dataOut) -> Vector Concatenate/37
  Weight Storage37/1(Out1) -> adder37/1(In1)
  adder37/1(dataOut) -> Vector Concatenate/38
  Weight Storage38/1(Out1) -> adder38/1(In1)
  adder38/1(dataOut) -> Vector Concatenate/39
  Weight Storage39/1(Out1) -> adder39/1(In1)
  adder39/1(dataOut) -> Vector Concatenate/40
  Weight Storage40/1(Out1) -> adder40/1(In1)
  adder40/1(dataOut) -> Vector Concatenate/41
  Weight Storage41/1(Out1) -> adder41/1(In1)
  adder41/1(dataOut) -> Vector Concatenate/42
  Weight Storage42/1(Out1) -> adder42/1(In1)
  adder42/1(dataOut) -> Vector Concatenate/43
  Weight Storage43/1(Out1) -> adder43/1(In1)
  adder43/1(dataOut) -> Vector Concatenate/44
  Weight Storage44/1(Out1) -> adder44/1(In1)
  adder44/1(dataOut) -> Vector Concatenate/45
  Weight Storage45/1(Out1) -> adder45/1(In1)
  adder45/1(dataOut) -> Vector Concatenate/46
  Weight Storage46/1(Out1) -> adder46/1(In1)
  adder46/1(dataOut) -> Vector Concatenate/47
  Weight Storage47/1(Out1) -> adder47/1(In1)
  adder47/1(dataOut) -> Vector Concatenate/48
  Weight Storage48/1(Out1) -> adder48/1(In1)
  adder48/1(dataOut) -> Vector Concatenate/49
  Weight Storage49/1(Out1) -> adder49/1(In1)
  adder49/1(dataOut) -> Vector Concatenate/50
  Weight Storage50/1(Out1) -> adder50/1(In1)
  adder50/1(dataOut) -> Vector Concatenate/51
  Weight Storage51/1(Out1) -> adder51/1(In1)
  adder51/1(dataOut) -> Vector Concatenate/52
  Weight Storage52/1(Out1) -> adder52/1(In1)
  adder52/1(dataOut) -> Vector Concatenate/53
  Weight Storage53/1(Out1) -> adder53/1(In1)
  adder53/1(dataOut) -> Vector Concatenate/54
  Weight Storage54/1(Out1) -> adder54/1(In1)
  adder54/1(dataOut) -> Vector Concatenate/55
  Weight Storage55/1(Out1) -> adder55/1(In1)
  adder55/1(dataOut) -> Vector Concatenate/56
  Weight Storage56/1(Out1) -> adder56/1(In1)
  adder56/1(dataOut) -> Vector Concatenate/57
  Weight Storage57/1(Out1) -> adder57/1(In1)
  adder57/1(dataOut) -> Vector Concatenate/58
  Weight Storage58/1(Out1) -> adder58/1(In1)
  adder58/1(dataOut) -> Vector Concatenate/59
  Weight Storage59/1(Out1) -> adder59/1(In1)
  adder59/1(dataOut) -> Vector Concatenate/60
  Weight Storage60/1(Out1) -> adder60/1(In1)
  adder60/1(dataOut) -> Vector Concatenate/61
  Weight Storage61/1(Out1) -> adder61/1(In1)
  adder61/1(dataOut) -> Vector Concatenate/62
  Weight Storage62/1(Out1) -> adder62/1(In1)
  adder62/1(dataOut) -> Vector Concatenate/63
  Weight Storage63/1(Out1) -> adder63/1(In1)
  adder63/1(dataOut) -> Vector Concatenate/64
  Weight Storage64/1(Out1) -> adder64/1(In1)
  adder64/1(dataOut) -> Vector Concatenate/65
  Weight Storage65/1(Out1) -> adder65/1(In1)
  adder65/1(dataOut) -> Vector Concatenate/66
  Weight Storage66/1(Out1) -> adder66/1(In1)
  adder66/1(dataOut) -> Vector Concatenate/67
  Weight Storage67/1(Out1) -> adder67/1(In1)
  adder67/1(dataOut) -> Vector Concatenate/68
  Weight Storage68/1(Out1) -> adder68/1(In1)
  adder68/1(dataOut) -> Vector Concatenate/69
  Weight Storage69/1(Out1) -> adder69/1(In1)
  adder69/1(dataOut) -> Vector Concatenate/70
  Weight Storage70/1(Out1) -> adder70/1(In1)
  adder70/1(dataOut) -> Vector Concatenate/71
  Weight Storage71/1(Out1) -> adder71/1(In1)
  adder71/1(dataOut) -> Vector Concatenate/72
  Weight Storage72/1(Out1) -> adder72/1(In1)
  adder72/1(dataOut) -> Vector Concatenate/73
  Weight Storage73/1(Out1) -> adder73/1(In1)
  adder73/1(dataOut) -> Vector Concatenate/74
  Weight Storage74/1(Out1) -> adder74/1(In1)
  adder74/1(dataOut) -> Vector Concatenate/75
  Weight Storage75/1(Out1) -> adder75/1(In1)
  adder75/1(dataOut) -> Vector Concatenate/76
  Weight Storage76/1(Out1) -> adder76/1(In1)
  adder76/1(dataOut) -> Vector Concatenate/77
  Weight Storage77/1(Out1) -> adder77/1(In1)
  adder77/1(dataOut) -> Vector Concatenate/78
  Weight Storage78/1(Out1) -> adder78/1(In1)
  adder78/1(dataOut) -> Vector Concatenate/79
  Weight Storage79/1(Out1) -> adder79/1(In1)
  adder79/1(dataOut) -> Vector Concatenate/80
  Weight Storage80/1(Out1) -> adder80/1(In1)
  adder80/1(dataOut) -> Vector Concatenate/81
  Weight Storage81/1(Out1) -> adder81/1(In1)
  adder81/1(dataOut) -> Vector Concatenate/82
  Weight Storage82/1(Out1) -> adder82/1(In1)
  adder82/1(dataOut) -> Vector Concatenate/83
  Weight Storage83/1(Out1) -> adder83/1(In1)
  adder83/1(dataOut) -> Vector Concatenate/84
  Weight Storage84/1(Out1) -> adder84/1(In1)
  adder84/1(dataOut) -> Vector Concatenate/85
  Weight Storage85/1(Out1) -> adder85/1(In1)
  adder85/1(dataOut) -> Vector Concatenate/86
  Weight Storage86/1(Out1) -> adder86/1(In1)
  adder86/1(dataOut) -> Vector Concatenate/87
  Weight Storage87/1(Out1) -> adder87/1(In1)
  adder87/1(dataOut) -> Vector Concatenate/88
  Weight Storage88/1(Out1) -> adder88/1(In1)
  adder88/1(dataOut) -> Vector Concatenate/89
  Weight Storage89/1(Out1) -> adder89/1(In1)
  adder89/1(dataOut) -> Vector Concatenate/90
  Weight Storage90/1(Out1) -> adder90/1(In1)
  adder90/1(dataOut) -> Vector Concatenate/91
  Weight Storage91/1(Out1) -> adder91/1(In1)
  adder91/1(dataOut) -> Vector Concatenate/92
  Weight Storage92/1(Out1) -> adder92/1(In1)
  adder92/1(dataOut) -> Vector Concatenate/93
  Weight Storage93/1(Out1) -> adder93/1(In1)
  adder93/1(dataOut) -> Vector Concatenate/94
  Weight Storage94/1(Out1) -> adder94/1(In1)
  adder94/1(dataOut) -> Vector Concatenate/95
  Weight Storage95/1(Out1) -> adder95/1(In1)
  adder95/1(dataOut) -> Vector Concatenate/96
  Weight Storage96/1(Out1) -> adder96/1(In1)
  adder96/1(dataOut) -> Vector Concatenate/97
  Weight Storage97/1(Out1) -> adder97/1(In1)
  adder97/1(dataOut) -> Vector Concatenate/98
  Weight Storage98/1(Out1) -> adder98/1(In1)
  adder98/1(dataOut) -> Vector Concatenate/99
  Weight Storage99/1(Out1) -> adder99/1(In1)
  adder99/1(dataOut) -> Vector Concatenate/100
  Weight Storage100/1(Out1) -> adder100/1(In1)
  adder100/1(dataOut) -> Vector Concatenate/101
  Weight Storage101/1(Out1) -> adder101/1(In1)
  adder101/1(dataOut) -> Vector Concatenate/102
  Weight Storage102/1(Out1) -> adder102/1(In1)
  adder102/1(dataOut) -> Vector Concatenate/103
  Weight Storage103/1(Out1) -> adder103/1(In1)
  adder103/1(dataOut) -> Vector Concatenate/104
  Weight Storage104/1(Out1) -> adder104/1(In1)
  adder104/1(dataOut) -> Vector Concatenate/105
  Weight Storage105/1(Out1) -> adder105/1(In1)
  adder105/1(dataOut) -> Vector Concatenate/106
  Weight Storage106/1(Out1) -> adder106/1(In1)
  adder106/1(dataOut) -> Vector Concatenate/107
  Weight Storage107/1(Out1) -> adder107/1(In1)
  adder107/1(dataOut) -> Vector Concatenate/108
  Weight Storage108/1(Out1) -> adder108/1(In1)
  adder108/1(dataOut) -> Vector Concatenate/109
  Weight Storage109/1(Out1) -> adder109/1(In1)
  adder109/1(dataOut) -> Vector Concatenate/110
  Weight Storage110/1(Out1) -> adder110/1(In1)
  adder110/1(dataOut) -> Vector Concatenate/111
  Weight Storage111/1(Out1) -> adder111/1(In1)
  adder111/1(dataOut) -> Vector Concatenate/112
  Weight Storage112/1(Out1) -> adder112/1(In1)
  adder112/1(dataOut) -> Vector Concatenate/113
  Weight Storage113/1(Out1) -> adder113/1(In1)
  adder113/1(dataOut) -> Vector Concatenate/114
  Weight Storage114/1(Out1) -> adder114/1(In1)
  adder114/1(dataOut) -> Vector Concatenate/115
  Weight Storage115/1(Out1) -> adder115/1(In1)
  adder115/1(dataOut) -> Vector Concatenate/116
  Weight Storage116/1(Out1) -> adder116/1(In1)
  adder116/1(dataOut) -> Vector Concatenate/117
  Weight Storage117/1(Out1) -> adder117/1(In1)
  adder117/1(dataOut) -> Vector Concatenate/118
  Weight Storage118/1(Out1) -> adder118/1(In1)
  adder118/1(dataOut) -> Vector Concatenate/119
  Weight Storage119/1(Out1) -> adder119/1(In1)
  adder119/1(dataOut) -> Vector Concatenate/120
  Weight Storage120/1(Out1) -> adder120/1(In1)
  adder120/1(dataOut) -> Vector Concatenate/121
  Weight Storage121/1(Out1) -> adder121/1(In1)
  adder121/1(dataOut) -> Vector Concatenate/122
  Weight Storage122/1(Out1) -> adder122/1(In1)
  adder122/1(dataOut) -> Vector Concatenate/123
  Weight Storage123/1(Out1) -> adder123/1(In1)
  adder123/1(dataOut) -> Vector Concatenate/124
  Weight Storage124/1(Out1) -> adder124/1(In1)
  adder124/1(dataOut) -> Vector Concatenate/125
  Weight Storage125/1(Out1) -> adder125/1(In1)
  adder125/1(dataOut) -> Vector Concatenate/126
  Weight Storage126/1(Out1) -> adder126/1(In1)
  adder126/1(dataOut) -> Vector Concatenate/127
  Weight Storage127/1(Out1) -> adder127/1(In1)
  adder127/1(dataOut) -> Vector Concatenate/128
  Delay/1 -> adder126/2(In2), adder127/2(In2), adder125/2(In2), adder124/2(In2), adder123/2(In2), adder122/2(In2), adder121/2(In2), adder120/2(In2), adder119/2(In2), adder118/2(In2), adder117/2(In2), adder116/2(In2), adder115/2(In2), adder114/2(In2), adder113/2(In2), adder112/2(In2), adder111/2(In2), adder110/2(In2), adder109/2(In2), adder108/2(In2), adder107/2(In2), adder106/2(In2), adder105/2(In2), adder104/2(In2), adder103/2(In2), adder102/2(In2), adder101/2(In2), adder100/2(In2), adder99/2(In2), adder98/2(In2), adder97/2(In2), adder96/2(In2), adder95/2(In2), adder94/2(In2), adder93/2(In2), adder92/2(In2), adder91/2(In2), adder90/2(In2), adder89/2(In2), adder88/2(In2), adder87/2(In2), adder86/2(In2), adder85/2(In2), adder84/2(In2), adder83/2(In2), adder82/2(In2), adder81/2(In2), adder80/2(In2), adder79/2(In2), adder78/2(In2), adder77/2(In2), adder76/2(In2), adder75/2(In2), adder74/2(In2), adder73/2(In2), adder72/2(In2), adder71/2(In2), adder70/2(In2), adder69/2(In2), adder68/2(In2), adder67/2(In2), adder65/2(In2), adder66/2(In2), adder64/2(In2), adder63/2(In2), adder62/2(In2), adder61/2(In2), adder60/2(In2), adder59/2(In2), adder58/2(In2), adder57/2(In2), adder56/2(In2), adder55/2(In2), adder54/2(In2), adder53/2(In2), adder52/2(In2), adder51/2(In2), adder50/2(In2), adder49/2(In2), adder48/2(In2), adder47/2(In2), adder46/2(In2), adder45/2(In2), adder44/2(In2), adder43/2(In2), adder42/2(In2), adder41/2(In2), adder40/2(In2), adder39/2(In2), adder38/2(In2), adder37/2(In2), adder36/2(In2), adder35/2(In2), adder34/2(In2), adder33/2(In2), adder32/2(In2), adder31/2(In2), adder30/2(In2), adder29/2(In2), adder28/2(In2), adder27/2(In2), adder26/2(In2), adder25/2(In2), adder24/2(In2), adder23/2(In2), adder22/2(In2), adder21/2(In2), adder20/2(In2), adder19/2(In2), adder18/2(In2), adder17/2(In2), adder16/2(In2), adder15/2(In2), adder14/2(In2), adder13/2(In2), adder12/2(In2), adder11/2(In2), adder10/2(In2), adder9/2(In2), adder8/2(In2), adder7/2(In2), adder6/2(In2), adder5/2(In2), adder4/2(In2), adder3/2(In2), adder2/2(In2), adder1/2(In2), adder 0/2(In2)  "sampleIn"

== system model_cnn/HDL CNN Model/Dense Layer 2/Dense Layer 2 ==
  note: make a look up table with matlab function block for weight storage - make sure to map to BRAMs
  dataIn : Inport
  validIn : Inport  Port=2
  Delay : Delay  DelayLength=1
  Delay1 : Delay  DelayLength=1
  HDL Counter : hdlsllib/Sources/HDL Counter  Commented=on  CountType=Count limited  CountInit=0  CountStep=1  CountMax=(1984*124)-1  CountFromType=Initial value  CountFrom=0  CountResetPort=off  CountLoadPort=off  CountEnbPort=on  CountDirPort=off  CountDataType=Unsigned  CountWordLen=ceil(log2(1984*124))  CountFracLen=0  CountSampTime=1
  HDL Counter1 : hdlsllib/Sources/HDL Counter  CountType=Count limited  CountInit=0  CountStep=1  CountMax=128-1  CountFromType=Initial value  CountFrom=0  CountResetPort=off  CountLoadPort=off  CountEnbPort=on  CountDirPort=off  CountDataType=Unsigned  CountWordLen=ceil(log2(128))  CountFracLen=0  CountSampTime=1
  Multiply-Accumulate : hdlsllib/HDL Operations/Multiply-Accumulate  Commented=on  opMode=Streaming - using Number of Samples  initValueSetting=Dialog  initValue=0  initValueSetting2=Dialog  initValue2=0  initValueSetting3=Dialog  initValue3=0  num_samples=1984  RndMeth2=Floor  RndMeth3=Floor  datatype2=Inherit: Inherit via back propagation  datatype3=fixdt(1,16,10)  validOut=on  endInandOut=on  startOut=on  countOut=on  dim=-1  DoSatur=off  parallel=off
      settings: SourceProductBaseCode=SL
  Terminator : Terminator  Commented=on
  Terminator1 : Terminator  Commented=on
  Terminator{2..8} (7 alike) : Terminator
  Vector Concatenate : Concatenate  NumInputs=8
  Weight Storage 0 : Subsystem  mask{dim=1}
      mask prompts: dim "Filter Selection"
  Weight Storage 1 : Subsystem  mask{dim=2}
      mask prompts: dim "Filter Selection"
  Weight Storage 2 : Subsystem  mask{dim=3}
      mask prompts: dim "Filter Selection"
  Weight Storage 3 : Subsystem  mask{dim=4}
      mask prompts: dim "Filter Selection"
  Weight Storage 4 : Subsystem  mask{dim=5}
      mask prompts: dim "Filter Selection"
  Weight Storage 5 : Subsystem  mask{dim=6}
      mask prompts: dim "Filter Selection"
  Weight Storage 6 : Subsystem  mask{dim=7}
      mask prompts: dim "Filter Selection"
  Weight Storage 7 : Subsystem  mask{dim=8}
      mask prompts: dim "Filter Selection"
  adder 0 : Subsystem
  adder 1 : Subsystem
  adder 2 : Subsystem
  adder 3 : Subsystem
  adder 4 : Subsystem
  adder 5 : Subsystem
  adder 6 : Subsystem
  adder 7 : Subsystem
  weight storage : Subsystem  Commented=on
  dataOut : Outport
  validOut : Outport  Port=2
  wires:
  Multiply-Accumulate/4 -> Terminator1/1
  Multiply-Accumulate/2 -> ?
  Multiply-Accumulate/1 -> ?
  ? -> HDL Counter/1, Multiply-Accumulate/3
  ? -> Multiply-Accumulate/1
  HDL Counter/1 -> weight storage/1(count_in)
  Multiply-Accumulate/3 -> Terminator/1
  weight storage/1(Out1) -> Multiply-Accumulate/2
  adder 0/1(dataOut) -> Vector Concatenate/1
  dataIn/1 -> Delay/1
  validIn/1 -> HDL Counter1/1, Delay1/1
  HDL Counter1/1 -> Weight Storage 7/1(count_Weights), Weight Storage 6/1(count_Weights), Weight Storage 5/1(count_Weights), Weight Storage 4/1(count_Weights), Weight Storage 3/1(count_Weights), Weight Storage 2/1(count_Weights), Weight Storage 1/1(count_Weights), Weight Storage 0/1(count_Weights)  "count_Weights"
  Weight Storage 0/1(Out1) -> adder 0/1(In1)
  adder 0/2(validOut) -> validOut/1
  Weight Storage 1/1(Out1) -> adder 1/1(In1)
  Weight Storage 2/1(Out1) -> adder 2/1(In1)
  Weight Storage 3/1(Out1) -> adder 3/1(In1)
  Weight Storage 4/1(Out1) -> adder 4/1(In1)
  Weight Storage 5/1(Out1) -> adder 5/1(In1)
  Weight Storage 6/1(Out1) -> adder 6/1(In1)
  Delay/1 -> adder 1/2(In2), adder 2/2(In2), adder 3/2(In2), adder 4/2(In2), adder 5/2(In2), adder 7/2(In2), adder 6/2(In2), adder 0/2(In2)
  Weight Storage 7/1(Out1) -> adder 7/1(In1)
  Delay1/1 -> adder 1/3(In3), adder 2/3(In3), adder 3/3(In3), adder 4/3(In3), adder 5/3(In3), adder 7/3(In3), adder 6/3(In3), adder 0/3(In3)
  adder 1/2(validOut) -> Terminator2/1
  adder 2/2(validOut) -> Terminator3/1
  adder 3/2(validOut) -> Terminator4/1
  adder 4/2(validOut) -> Terminator5/1
  adder 5/2(validOut) -> Terminator6/1
  adder 6/2(validOut) -> Terminator7/1
  adder 7/2(validOut) -> Terminator8/1
  adder 1/1(dataOut) -> Vector Concatenate/2
  adder 2/1(dataOut) -> Vector Concatenate/3
  adder 3/1(dataOut) -> Vector Concatenate/4
  adder 4/1(dataOut) -> Vector Concatenate/5
  adder 5/1(dataOut) -> Vector Concatenate/6
  adder 6/1(dataOut) -> Vector Concatenate/7
  adder 7/1(dataOut) -> Vector Concatenate/8
  Vector Concatenate/1 -> dataOut/1

== system model_cnn/HDL CNN Model/Conv Layer 1/Layer 1 Mat-Vec Multiplier/Weight Storage 0 ==
  count_Weights : Inport
  Constant : Constant  Value=0  OutDataTypeStr=gemm_wconv1.numerictype  SampleTime=-1
  Constant1 : Constant  Value=false  SampleTime=-1
  Single Port RAM System : hdlsllib/HDL RAMs/Single Port RAM System  RAMType=Single port  WriteOutputValue=New data  RAMInitialValue=[gemm_wconv1(dim,:),zeros(1,4-3)]  SimulateUsing=Code generation
      settings: SourceProductBaseCode=SL
  Out1 : Outport
  wires:
  count_Weights/1 -> Single Port RAM System/2
  Constant1/1 -> Single Port RAM System/3
  Constant/1 -> Single Port RAM System/1
  Single Port RAM System/1 -> Out1/1

== system model_cnn/HDL CNN Model/Conv Layer 1/Layer 1 Mat-Vec Multiplier/Weight Storage1 ==
  count_Weights : Inport
  Constant : Constant  Value=0  OutDataTypeStr=gemm_wconv1.numerictype  SampleTime=-1
  Constant1 : Constant  Value=false  SampleTime=-1
  Single Port RAM System : hdlsllib/HDL RAMs/Single Port RAM System  RAMType=Single port  WriteOutputValue=New data  RAMInitialValue=[gemm_wconv1(dim,:),zeros(1,4-3)]  SimulateUsing=Code generation
      settings: SourceProductBaseCode=SL
  Out1 : Outport
  wires:
  Single Port RAM System/1 -> Out1/1
  Constant/1 -> Single Port RAM System/1
  Constant1/1 -> Single Port RAM System/3
  count_Weights/1 -> Single Port RAM System/2

== system model_cnn/HDL CNN Model/Conv Layer 1/Layer 1 Mat-Vec Multiplier/Weight Storage10 ==
  count_Weights : Inport
  Constant : Constant  Value=0  OutDataTypeStr=gemm_wconv1.numerictype  SampleTime=-1
  Constant1 : Constant  Value=false  SampleTime=-1
  Single Port RAM System : hdlsllib/HDL RAMs/Single Port RAM System  RAMType=Single port  WriteOutputValue=New data  RAMInitialValue=[gemm_wconv1(dim,:),zeros(1,4-3)]  SimulateUsing=Code generation
      settings: SourceProductBaseCode=SL
  Out1 : Outport
  wires:
  Single Port RAM System/1 -> Out1/1
  Constant/1 -> Single Port RAM System/1
  Constant1/1 -> Single Port RAM System/3
  count_Weights/1 -> Single Port RAM System/2

== system model_cnn/HDL CNN Model/Conv Layer 1/Layer 1 Mat-Vec Multiplier/Weight Storage11 ==
  count_Weights : Inport
  Constant : Constant  Value=0  OutDataTypeStr=gemm_wconv1.numerictype  SampleTime=-1
  Constant1 : Constant  Value=false  SampleTime=-1
  Single Port RAM System : hdlsllib/HDL RAMs/Single Port RAM System  RAMType=Single port  WriteOutputValue=New data  RAMInitialValue=[gemm_wconv1(dim,:),zeros(1,4-3)]  SimulateUsing=Code generation
      settings: SourceProductBaseCode=SL
  Out1 : Outport
  wires:
  Single Port RAM System/1 -> Out1/1
  Constant/1 -> Single Port RAM System/1
  Constant1/1 -> Single Port RAM System/3
  count_Weights/1 -> Single Port RAM System/2

== system model_cnn/HDL CNN Model/Conv Layer 1/Layer 1 Mat-Vec Multiplier/Weight Storage12 ==
  count_Weights : Inport
  Constant : Constant  Value=0  OutDataTypeStr=gemm_wconv1.numerictype  SampleTime=-1
  Constant1 : Constant  Value=false  SampleTime=-1
  Single Port RAM System : hdlsllib/HDL RAMs/Single Port RAM System  RAMType=Single port  WriteOutputValue=New data  RAMInitialValue=[gemm_wconv1(dim,:),zeros(1,4-3)]  SimulateUsing=Code generation
      settings: SourceProductBaseCode=SL
  Out1 : Outport
  wires:
  Single Port RAM System/1 -> Out1/1
  Constant/1 -> Single Port RAM System/1
  Constant1/1 -> Single Port RAM System/3
  count_Weights/1 -> Single Port RAM System/2
